simulink model "sampleModel106"  (R2022a)
settings: Solver=VariableStepAuto  StartTime=0.0  StopTime=10.0  RelTol=1e-3
undefined symbols (not defined in the file): DiscIntNeverNeededParam, magnitude, Newton, Raphson
libraries: simulink x379, slpidlib x89
(part 13 of 16)

== system sampleModel106/cfblk83/cfblk12/cfblk12/cfblk10 ==
  cfblk1 : Inport
  cfblk10 : Inport  Port=2
  cfblk11 : Inport  Port=3
  cfblk12 : Inport  Port=4
  cfblk13 : Inport  Port=5
  cfblk3 : DiscreteStateSpace
  cfblk4 : simulink/Discrete/Transfer Fcn Lead or Lag  PoleZ=0.95  ZeroZ=0.75  ICPrevOutput=0.0  ICPrevInput=0.0  DoSatur=off
      settings: SourceProductBaseCode=SL
  cfblk5 : ComplexToMagnitudeAngle
  cfblk6 : Reshape
  cfblk7 : PermuteDimensions
  cfblk8 : Signum
  cfblk9 : Constant  Value=[-735984474.100550]  SampleTime=1
  cfblk2 : Outport
  cfblk14 : Outport  Port=2
  cfblk15 : Outport  Port=3
  wires:
  cfblk6/1 -> cfblk8/1
  cfblk8/1 -> cfblk3/1
  cfblk5/1 -> cfblk15/1
  cfblk3/1 -> cfblk5/1
  cfblk10/1 -> cfblk7/1
  cfblk7/1 -> cfblk6/1
  cfblk13/1 -> cfblk4/1
  cfblk9/1 -> cfblk2/1
  cfblk12/1 -> cfblk14/1

== system sampleModel106/cfblk83/cfblk12/cfblk12/cfblk11 ==
  cfblk1 : Inport
  cfblk11 : Inport  Port=2
  cfblk12 : Inport  Port=3
  cfblk10 : Constant  Value=[-348173001.781500]  SampleTime=1
  cfblk3 : simulink/Discrete/Difference  ICPrevInput=0.0  OutMin=[]  OutMax=[]  OutDataTypeStr=Inherit: Inherit via back propagation  OutDataType=fixdt(1, 16)  OutScaling=2^-10  DoSatur=off
  cfblk4 : simulink/Discrete/Transfer Fcn First Order  PoleZ=0.95  ICPrevOutput=0.0  DoSatur=off
  cfblk5 : slpidlib/PID Controller  Controller=PID  Form=Parallel  TimeDomain=Discrete-time  UseExternalTs=off  SampleTime=1  IntegratorMethod=Forward Euler  FilterMethod=Forward Euler  ControllerParametersSource=internal  P=1  I=1  UseKiTs=off  D=0  N=100  UseFilter=on  TunerSelectOption=Transfer Function Based (PID Tuner App)  InitialConditionSource=internal  InitialConditionForIntegrator=0  InitialConditionForFilter=0  DifferentiatorICPrevScaledInput=0  ExternalReset=none  TrackingMode=off  Kt=1  LimitOutput=off  SatLimitsSource=internal  UpperSaturationLimit=inf  LowerSaturationLimit=-inf  LinearizeAsGain=off  AntiWindupMode=none  Kb=1  POutMin=[]  POutMax=[]  IOutMin=[]  IOutMax=[]  DOutMin=[]  DOutMax=[]  NOutMin=[]  NOutMax=[]  SumOutMin=[]  SumOutMax=[]  SaturationOutMin=[]  SaturationOutMax=[]  PParamMin=[]  PParamMax=[]  IParamMin=[]  IParamMax=[]  DParamMin=[]  DParamMax=[]  NParamMin=[]  NParamMax=[]  KbParamMin=[]  KbParamMax=[]  KtParamMin=[]  KtParamMax=[]  KbOutMin=[]  KbOutMax=[]  KtOutMin=[]  KtOutMax=[]  IntegratorOutMin=[]  IntegratorOutMax=[]  FilterOutMin=[]  FilterOutMax=[]  SumI1OutMin=[]  SumI1OutMax=[]  SumI2OutMin=[]  SumI2OutMax=[]  SumI3OutMin=[]  SumI3OutMax=[]  SumI4OutMin=[]  SumI4OutMax=[]  SumDOutMin=[]  SumDOutMax=[]  DifferentiatorOutMin=[]  DifferentiatorOutMax=[]  FilterDiffOutCoefMin=[]  FilterDiffOutCoefMax=[]  ReciprocalOutMin=[]  ReciprocalOutMax=[]  SumDenOutMin=[]  SumDenOutMax=[]  SumNumOutMin=[]  SumNumOutMax=[]  DivideOutMin=[]  DivideOutMax=[]  UdiffTsProdOutMin=[]  UdiffTsProdOutMax=[]  NTsProdOutMin=[]  NTsProdOutMax=[]  UintegralTsProdOutMin=[]  UintegralTsProdOutMax=[]  UngainTsProdOutMin=[]  UngainTsProdOutMax=[]  IntegratorContinuousStateAttributes=''  IntegratorStateMustResolveToSignalObject=off  IntegratorRTWStateStorageClass=Auto  FilterContinuousStateAttributes=''  FilterStateMustResolveToSignalObject=off  FilterRTWStateStorageClass=Auto  ParallelPVariant=InternalParameters  IdealPVariant=Disabled  IVariant=InternalParameters  DVariant=InternalParameters  IntegratorVariant=Discrete  SatVariant=Disabled  AWVariant=Passthrough  PCopyVariant=Disabled  TRVariant=Disabled  FdbkBlocksVariant=Forward  IdealPFdbkVariant=Disabled  SatFdbkVariant=Disabled  DerivativeFilterVariant=ForwardEulerFilter  NVariant=InternalParameters  NCopyVariant=Disabled  FilterICVariant=InternalICsFilter  IntegratorICVariant=InternalICs  ExternalResetVariant=Disabled  TRSumVariant=Passthrough  SumFdbkVariant=Disabled  SumVariant=Sum_PID  TsampFilterVariant=InternalTs  TsampNgainVariant=Passthrough  TsampIntegralVariant=Passthrough  ExternalSaturationOutDataTypeStr=Inherit: Same as second input  aMode=0
  cfblk6 : Rounding
  cfblk7 : Signum
  cfblk8 : Sqrt  Operator=rSqrt  AlgorithmType=Newton-Raphson
  cfblk9 : Constant  Value=[207257755.323865]  SampleTime=1
  cfblk2 : Outport
  wires:
  cfblk9/1 -> cfblk3/1
  cfblk7/1 -> cfblk2/1
  cfblk11/1 -> cfblk5/1
  cfblk10/1 -> cfblk7/1
  cfblk12/1 -> cfblk8/1
  cfblk6/1 -> cfblk4/1
  cfblk1/1 -> cfblk6/1

== system sampleModel106/cfblk83/cfblk12/cfblk13/cfblk10 ==
  cfblk1 : Inport
  cfblk10 : Sum  Inputs=--
  cfblk11 : Sin  TimeSource=Use external signal  SampleTime=0
  cfblk12 : Squeeze
  cfblk13 : Constant  Value=[-66310425.135306]  SampleTime=1
  cfblk14 : Constant  Value=[-311313699.679596]  SampleTime=1
  cfblk3 : DiscreteTransferFcn  SampleTime=1
  cfblk4 : slpidlib/PID Controller  Controller=PID  Form=Parallel  TimeDomain=Discrete-time  UseExternalTs=off  SampleTime=1  IntegratorMethod=Forward Euler  FilterMethod=Forward Euler  ControllerParametersSource=internal  P=1  I=1  UseKiTs=off  D=0  N=100  UseFilter=on  TunerSelectOption=Transfer Function Based (PID Tuner App)  InitialConditionSource=internal  InitialConditionForIntegrator=0  InitialConditionForFilter=0  DifferentiatorICPrevScaledInput=0  ExternalReset=none  TrackingMode=off  Kt=1  LimitOutput=off  SatLimitsSource=internal  UpperSaturationLimit=inf  LowerSaturationLimit=-inf  LinearizeAsGain=off  AntiWindupMode=none  Kb=1  POutMin=[]  POutMax=[]  IOutMin=[]  IOutMax=[]  DOutMin=[]  DOutMax=[]  NOutMin=[]  NOutMax=[]  SumOutMin=[]  SumOutMax=[]  SaturationOutMin=[]  SaturationOutMax=[]  PParamMin=[]  PParamMax=[]  IParamMin=[]  IParamMax=[]  DParamMin=[]  DParamMax=[]  NParamMin=[]  NParamMax=[]  KbParamMin=[]  KbParamMax=[]  KtParamMin=[]  KtParamMax=[]  KbOutMin=[]  KbOutMax=[]  KtOutMin=[]  KtOutMax=[]  IntegratorOutMin=[]  IntegratorOutMax=[]  FilterOutMin=[]  FilterOutMax=[]  SumI1OutMin=[]  SumI1OutMax=[]  SumI2OutMin=[]  SumI2OutMax=[]  SumI3OutMin=[]  SumI3OutMax=[]  SumI4OutMin=[]  SumI4OutMax=[]  SumDOutMin=[]  SumDOutMax=[]  DifferentiatorOutMin=[]  DifferentiatorOutMax=[]  FilterDiffOutCoefMin=[]  FilterDiffOutCoefMax=[]  ReciprocalOutMin=[]  ReciprocalOutMax=[]  SumDenOutMin=[]  SumDenOutMax=[]  SumNumOutMin=[]  SumNumOutMax=[]  DivideOutMin=[]  DivideOutMax=[]  UdiffTsProdOutMin=[]  UdiffTsProdOutMax=[]  NTsProdOutMin=[]  NTsProdOutMax=[]  UintegralTsProdOutMin=[]  UintegralTsProdOutMax=[]  UngainTsProdOutMin=[]  UngainTsProdOutMax=[]  IntegratorContinuousStateAttributes=''  IntegratorStateMustResolveToSignalObject=off  IntegratorRTWStateStorageClass=Auto  FilterContinuousStateAttributes=''  FilterStateMustResolveToSignalObject=off  FilterRTWStateStorageClass=Auto  ParallelPVariant=InternalParameters  IdealPVariant=Disabled  IVariant=InternalParameters  DVariant=InternalParameters  IntegratorVariant=Discrete  SatVariant=Disabled  AWVariant=Passthrough  PCopyVariant=Disabled  TRVariant=Disabled  FdbkBlocksVariant=Forward  IdealPFdbkVariant=Disabled  SatFdbkVariant=Disabled  DerivativeFilterVariant=ForwardEulerFilter  NVariant=InternalParameters  NCopyVariant=Disabled  FilterICVariant=InternalICsFilter  IntegratorICVariant=InternalICs  ExternalResetVariant=Disabled  TRSumVariant=Passthrough  SumFdbkVariant=Disabled  SumVariant=Sum_PID  TsampFilterVariant=InternalTs  TsampNgainVariant=Passthrough  TsampIntegralVariant=Passthrough  ExternalSaturationOutDataTypeStr=Inherit: Same as second input  aMode=0
  cfblk5 : simulink/Discrete/Transfer Fcn First Order  PoleZ=0.95  ICPrevOutput=0.0  DoSatur=off
  cfblk6 : Signum
  cfblk7 : Sum  Inputs=-+
  cfblk8 : UnaryMinus
  cfblk9 : Math  Operator=conj
  cfblk2 : Outport
  cfblk15 : Outport  Port=2
  cfblk16 : Outport  Port=3
  cfblk17 : Outport  Port=4
  wires:
  cfblk5/1 -> cfblk17/1
  cfblk7/1 -> cfblk15/1
  cfblk14/1 -> cfblk6/1
  cfblk13/1 -> cfblk4/1, cfblk11/1
  cfblk11/1 -> cfblk5/1, cfblk10/2
  cfblk1/1 -> cfblk10/1, cfblk9/1
  cfblk10/1 -> cfblk3/1
  cfblk9/1 -> cfblk7/1
  cfblk8/1 -> cfblk2/1
  cfblk6/1 -> cfblk7/2
  cfblk3/1 -> cfblk16/1
  cfblk4/1 -> cfblk12/1
  cfblk12/1 -> cfblk8/1

== system sampleModel106/cfblk83/cfblk12/cfblk13/cfblk8 ==
  cfblk1 : Inport
  cfblk13 : Inport  Port=2
  cfblk14 : Inport  Port=3
  cfblk10 : Constant  Value=[-221630629.444218]  SampleTime=1
  cfblk11 : Constant  Value=[651188913.954120]  SampleTime=1
  cfblk12 : Constant  Value=[-519214434.322099]  SampleTime=1
  cfblk3 : DiscreteTransferFcn  SampleTime=1
  cfblk4 : Delay  DelayLengthSource=Input port  SampleTime=1
      settings: InputPortMap=u0,p1
  cfblk5 : DiscreteFilter  SampleTime=1
  cfblk6 : slpidlib/PID Controller  Controller=PID  Form=Parallel  TimeDomain=Discrete-time  UseExternalTs=off  SampleTime=1  IntegratorMethod=Forward Euler  FilterMethod=Forward Euler  ControllerParametersSource=internal  P=1  I=1  UseKiTs=off  D=0  N=100  UseFilter=on  TunerSelectOption=Transfer Function Based (PID Tuner App)  InitialConditionSource=internal  InitialConditionForIntegrator=0  InitialConditionForFilter=0  DifferentiatorICPrevScaledInput=0  ExternalReset=none  TrackingMode=off  Kt=1  LimitOutput=off  SatLimitsSource=internal  UpperSaturationLimit=inf  LowerSaturationLimit=-inf  LinearizeAsGain=off  AntiWindupMode=none  Kb=1  POutMin=[]  POutMax=[]  IOutMin=[]  IOutMax=[]  DOutMin=[]  DOutMax=[]  NOutMin=[]  NOutMax=[]  SumOutMin=[]  SumOutMax=[]  SaturationOutMin=[]  SaturationOutMax=[]  PParamMin=[]  PParamMax=[]  IParamMin=[]  IParamMax=[]  DParamMin=[]  DParamMax=[]  NParamMin=[]  NParamMax=[]  KbParamMin=[]  KbParamMax=[]  KtParamMin=[]  KtParamMax=[]  KbOutMin=[]  KbOutMax=[]  KtOutMin=[]  KtOutMax=[]  IntegratorOutMin=[]  IntegratorOutMax=[]  FilterOutMin=[]  FilterOutMax=[]  SumI1OutMin=[]  SumI1OutMax=[]  SumI2OutMin=[]  SumI2OutMax=[]  SumI3OutMin=[]  SumI3OutMax=[]  SumI4OutMin=[]  SumI4OutMax=[]  SumDOutMin=[]  SumDOutMax=[]  DifferentiatorOutMin=[]  DifferentiatorOutMax=[]  FilterDiffOutCoefMin=[]  FilterDiffOutCoefMax=[]  ReciprocalOutMin=[]  ReciprocalOutMax=[]  SumDenOutMin=[]  SumDenOutMax=[]  SumNumOutMin=[]  SumNumOutMax=[]  DivideOutMin=[]  DivideOutMax=[]  UdiffTsProdOutMin=[]  UdiffTsProdOutMax=[]  NTsProdOutMin=[]  NTsProdOutMax=[]  UintegralTsProdOutMin=[]  UintegralTsProdOutMax=[]  UngainTsProdOutMin=[]  UngainTsProdOutMax=[]  IntegratorContinuousStateAttributes=''  IntegratorStateMustResolveToSignalObject=off  IntegratorRTWStateStorageClass=Auto  FilterContinuousStateAttributes=''  FilterStateMustResolveToSignalObject=off  FilterRTWStateStorageClass=Auto  ParallelPVariant=InternalParameters  IdealPVariant=Disabled  IVariant=InternalParameters  DVariant=InternalParameters  IntegratorVariant=Discrete  SatVariant=Disabled  AWVariant=Passthrough  PCopyVariant=Disabled  TRVariant=Disabled  FdbkBlocksVariant=Forward  IdealPFdbkVariant=Disabled  SatFdbkVariant=Disabled  DerivativeFilterVariant=ForwardEulerFilter  NVariant=InternalParameters  NCopyVariant=Disabled  FilterICVariant=InternalICsFilter  IntegratorICVariant=InternalICs  ExternalResetVariant=Disabled  TRSumVariant=Passthrough  SumFdbkVariant=Disabled  SumVariant=Sum_PID  TsampFilterVariant=InternalTs  TsampNgainVariant=Passthrough  TsampIntegralVariant=Passthrough  ExternalSaturationOutDataTypeStr=Inherit: Same as second input  aMode=0
  cfblk7 : Sum  Inputs=|++
  cfblk8 : DotProduct  OutDataTypeStr=Inherit: Inherit via internal rule
  cfblk9 : Constant  Value=[-97885654.836450]  SampleTime=1
  cfblk2 : Outport
  cfblk15 : Outport  Port=2
  cfblk16 : Outport  Port=3
  cfblk17 : Outport  Port=4
  wires:
  cfblk13/1 -> cfblk7/1
  cfblk9/1 -> cfblk5/1
  cfblk1/1 -> cfblk8/1
  cfblk11/1 -> cfblk7/2
  cfblk3/1 -> cfblk15/1
  cfblk7/1 -> cfblk8/2
  cfblk12/1 -> cfblk2/1
  cfblk14/1 -> cfblk16/1
  cfblk8/1 -> cfblk3/1
  cfblk4/1 -> cfblk17/1
  cfblk10/1 -> cfblk6/1
  cfblk6/1 -> cfblk4/1
  cfblk5/1 -> cfblk4/2

== system sampleModel106/cfblk83/cfblk12/cfblk13/cfblk9 ==
  cfblk1 : Inport
  cfblk13 : Inport  Port=2
  cfblk14 : Inport  Port=3
  cfblk15 : Inport  Port=4
  cfblk16 : Inport  Port=5
  cfblk10 : Product
  cfblk11 : Constant  Value=[-59332882.686168]  SampleTime=1
  cfblk12 : Constant  Value=[889332264.177902]  SampleTime=1
  cfblk3 : simulink/Discrete/Transfer Fcn Real Zero  ZeroZ=0.75  ICPrevInput=0.0  DoSatur=off
      settings: SourceProductBaseCode=SL
  cfblk4 : DiscreteStateSpace
  cfblk5 : Math  Operator=pow
  cfblk6 : Sum  Inputs=+
  cfblk7 : Squeeze
  cfblk8 : Sum  Inputs=+-
  cfblk9 : Reshape
  cfblk2 : Outport
  cfblk17 : Outport  Port=2
  wires:
  cfblk13/1 -> cfblk4/1
  cfblk8/1 -> cfblk6/1
  cfblk9/1 -> cfblk17/1
  cfblk4/1 -> cfblk8/1
  cfblk7/1 -> cfblk3/1
  cfblk11/1 -> cfblk9/1
  cfblk16/1 -> cfblk5/1
  cfblk1/1 -> cfblk5/2
  cfblk12/1 -> cfblk2/1
  cfblk15/1 -> cfblk7/1
  cfblk5/1 -> cfblk8/2
  cfblk14/1 -> cfblk10/1
  cfblk6/1 -> cfblk10/2

== system sampleModel106/cfblk83/cfblk13/cfblk11/cfblk9 ==
  cfblk1 : Inport
  cfblk12 : Inport  Port=2
  cfblk10 : Constant  Value=[979832863.962545]  SampleTime=1
  cfblk11 : Constant  Value=[551392504.886462]  SampleTime=1
  cfblk14 : Delay  SampleTime=1
  cfblk3 : Sum  Inputs=+
  cfblk4 : Assignment  DiagnosticForDimensions=Warning  IndexOptions=Index vector (dialog)  Indices=1  OutputSizes=1
  cfblk5 : Sqrt
  cfblk6 : Sqrt  Operator=rSqrt  AlgorithmType=Newton-Raphson
  cfblk7 : Squeeze
  cfblk8 : Constant  Value=[798337658.700192]  SampleTime=1
  cfblk9 : Constant  Value=[-485920315.300231]  SampleTime=1
  cfblk2 : Outport
  cfblk13 : Outport  Port=2
  wires:
  cfblk11/1 -> cfblk7/1
  cfblk7/1 -> cfblk13/1
  cfblk9/1 -> cfblk5/1
  cfblk10/1 -> cfblk6/1
  cfblk1/1 -> cfblk2/1
  cfblk8/1 -> cfblk4/1
  cfblk3/1 -> cfblk4/2
  cfblk4/1 -> cfblk14/1
  cfblk14/1 -> cfblk3/1

== system sampleModel106/cfblk83/cfblk13/cfblk12/cfblk5 ==
  cfblk1 : Inport
  cfblk11 : Inport  Port=2
  cfblk12 : Inport  Port=3
  cfblk13 : Inport  Port=4
  cfblk14 : Inport  Port=5
  cfblk15 : Inport  Port=6
  cfblk16 : Inport  Port=7
  cfblk10 : Constant  Value=[611025124.323310]  SampleTime=1
  cfblk18 : Delay  SampleTime=1
  cfblk3 : Delay  ShowEnablePort=on  SampleTime=1
      settings: InputPortMap=u0,e6
  cfblk4 : Sum  Inputs=-+
  cfblk5 : Signum
  cfblk6 : Product
  cfblk7 : ComplexToMagnitudeAngle
  cfblk8 : DotProduct  OutDataTypeStr=Inherit: Inherit via internal rule
  cfblk9 : Assignment  DiagnosticForDimensions=Warning  IndexOptions=Index vector (dialog)  Indices=1  OutputSizes=1
  cfblk2 : Outport
  cfblk17 : Outport  Port=2
  wires:
  cfblk15/1 -> cfblk3/1
  cfblk5/1 -> cfblk7/1
  cfblk6/1 -> cfblk4/1
  cfblk1/1 -> cfblk3/2
  cfblk8/1 -> cfblk2/1
  cfblk12/1 -> cfblk8/1
  cfblk13/1 -> cfblk17/1
  cfblk16/1 -> cfblk5/1
  cfblk10/1 -> cfblk4/2
  cfblk11/1 -> cfblk9/1
  cfblk3/1 -> cfblk6/2
  cfblk7/1 -> cfblk8/2
  cfblk4/1 -> cfblk9/2
  cfblk9/1 -> cfblk18/1
  cfblk18/1 -> cfblk6/1

== system sampleModel106/cfblk83/cfblk13/cfblk12/cfblk6 ==
  cfblk1 : Inport
  cfblk10 : Gain  Gain=[293098853.914123]
  cfblk11 : Gain  Gain=[-612575929.200624]
  cfblk12 : Gain  Gain=[945578202.855884]
  cfblk13 : Constant  Value=[-519498832.994828]  SampleTime=1
  cfblk16 : Delay  SampleTime=1
  cfblk3 : Delay  DelayLengthSource=Input port  SampleTime=1
      settings: InputPortMap=u0,p1
  cfblk4 : simulink/Discrete/Difference  ICPrevInput=0.0  OutMin=[]  OutMax=[]  OutDataTypeStr=Inherit: Inherit via back propagation  OutDataType=fixdt(1, 16)  OutScaling=2^-10  DoSatur=off
  cfblk5 : Delay  ShowEnablePort=on  SampleTime=1
      settings: InputPortMap=u0,e6
  cfblk6 : UnitDelay  HasFrameUpgradeWarning=on
  cfblk7 : Rounding
  cfblk8 : MinMax  Function=max
  cfblk9 : Polyval  Coefs=[ +2.081618890e-019, -1.441693666e-014, +4.719686976e-010, -8.536869453e-006, +1.621573104e-001, -8.087801117e+001 ]
  cfblk2 : Outport
  cfblk14 : Outport  Port=2
  cfblk15 : Outport  Port=3
  wires:
  cfblk6/1 -> cfblk9/1
  cfblk12/1 -> cfblk14/1
  cfblk1/1 -> cfblk3/1
  cfblk9/1 -> cfblk15/1, cfblk5/2
  cfblk7/1 -> cfblk6/1
  cfblk3/1 -> cfblk8/1
  cfblk10/1 -> cfblk7/1
  cfblk4/1 -> cfblk5/1
  cfblk8/1 -> cfblk11/1, cfblk12/1
  cfblk13/1 -> cfblk2/1, cfblk10/1
  cfblk11/1 -> cfblk4/1
  cfblk5/1 -> cfblk16/1
  cfblk16/1 -> cfblk3/2

== system sampleModel106/cfblk83/cfblk13/cfblk12/cfblk7 ==
  cfblk1 : Inport
  cfblk12 : Inport  Port=2
  cfblk13 : Inport  Port=3
  cfblk14 : Inport  Port=4
  cfblk15 : Inport  Port=5
  cfblk10 : Constant  Value=[931392199.249037]  SampleTime=1
  cfblk11 : Constant  Value=[718235558.917173]  SampleTime=1
  cfblk3 : Delay  SampleTime=1
  cfblk4 : DiscreteFilter  SampleTime=1
  cfblk5 : Rounding
  cfblk6 : DotProduct  OutDataTypeStr=Inherit: Inherit via internal rule
  cfblk7 : UnaryMinus
  cfblk8 : Trigonometry
  cfblk9 : Squeeze
  cfblk2 : Outport
  cfblk16 : Outport  Port=2
  wires:
  cfblk11/1 -> cfblk6/1
  cfblk5/1 -> cfblk4/1
  cfblk6/1 -> cfblk7/1
  cfblk14/1 -> cfblk5/1
  cfblk12/1 -> cfblk6/2
  cfblk13/1 -> cfblk9/1
  cfblk9/1 -> cfblk2/1
  cfblk15/1 -> cfblk3/1
  cfblk7/1 -> cfblk16/1
  cfblk3/1 -> cfblk8/1

== system sampleModel106/cfblk83/cfblk13/cfblk12/cfblk8 ==
  cfblk1 : Inport
  cfblk7 : Inport  Port=2
  cfblk8 : Inport  Port=3
  cfblk3 : Abs  SaturateOnIntegerOverflow=off
  cfblk4 : ComplexToMagnitudeAngle
  cfblk5 : Sum  Inputs=|++
  cfblk6 : Squeeze
  cfblk2 : Outport
  wires:
  cfblk5/1 -> cfblk2/1
  cfblk4/1 -> cfblk6/1
  cfblk1/1 -> cfblk5/1
  cfblk8/1 -> cfblk3/1
  cfblk6/1 -> cfblk5/2
  cfblk7/1 -> cfblk4/1

== system sampleModel106/cfblk83/cfblk13/cfblk13/cfblk8 ==
  cfblk1 : Inport
  cfblk10 : Inport  Port=2
  cfblk11 : Inport  Port=3
  cfblk3 : Trigonometry
  cfblk4 : Trigonometry
  cfblk5 : Trigonometry
  cfblk6 : Sin  TimeSource=Use external signal  SampleTime=0
  cfblk7 : Squeeze
  cfblk8 : Sum  Inputs=|++
  cfblk9 : Constant  Value=[938603763.562760]  SampleTime=1
  cfblk2 : Outport
  cfblk12 : Outport  Port=2
  wires:
  cfblk4/1 -> cfblk8/1
  cfblk3/1 -> cfblk6/1
  cfblk9/1 -> cfblk4/1
  cfblk6/1 -> cfblk12/1
  cfblk1/1 -> cfblk8/2
  cfblk11/1 -> cfblk5/1
  cfblk5/1 -> cfblk3/1
  cfblk10/1 -> cfblk7/1
  cfblk8/1 -> cfblk2/1

== system sampleModel106/cfblk83/cfblk13/cfblk13/cfblk9 ==
  cfblk1 : Inport
  cfblk11 : Inport  Port=2
  cfblk10 : Constant  Value=[825217161.468918]  SampleTime=1
  cfblk13 : Delay  SampleTime=1
  cfblk3 : UnitDelay  HasFrameUpgradeWarning=on
  cfblk4 : UnitDelay  HasFrameUpgradeWarning=on
  cfblk5 : DiscreteFir  SampleTime=1
  cfblk6 : simulink/Discrete/Transfer Fcn First Order  PoleZ=0.95  ICPrevOutput=0.0  DoSatur=off
  cfblk7 : ComplexToMagnitudeAngle
  cfblk8 : Sum  Inputs=+
  cfblk9 : Constant  Value=[262988150.516446]  SampleTime=1
  cfblk2 : Outport
  cfblk12 : Outport  Port=2
  wires:
  cfblk8/1 -> cfblk6/1
  cfblk10/1 -> cfblk8/1
  cfblk1/1 -> cfblk2/1
  cfblk9/1 -> cfblk12/1
  cfblk3/1 -> cfblk7/1
  cfblk7/1 -> cfblk4/1
  cfblk7/2 -> cfblk5/1
  cfblk4/1 -> cfblk13/1
  cfblk13/1 -> cfblk3/1

== system sampleModel106/cfblk84/cfblk10/cfblk10/cfblk10 ==
  cfblk1 : Inport
  cfblk6 : Inport  Port=2
  cfblk3 : UnitDelay  SampleTime=-1  HasFrameUpgradeWarning=on
  cfblk4 : Product  Inputs=*
  cfblk5 : DotProduct  OutDataTypeStr=Inherit: Inherit via internal rule
  cfblk2 : Outport
  cfblk7 : Outport  Port=2
  wires:
  cfblk4/1 -> cfblk2/1
  cfblk3/1 -> cfblk4/1, cfblk5/2
  cfblk6/1 -> cfblk3/1
  cfblk5/1 -> cfblk7/1
  cfblk1/1 -> cfblk5/1

== system sampleModel106/cfblk84/cfblk10/cfblk10/cfblk11 ==
  cfblk1 : Inport
  cfblk7 : Inport  Port=2
  cfblk3 : DiscreteFilter
  cfblk4 : Sum  Inputs=|++
  cfblk5 : Product  Inputs=*
  cfblk6 : Sqrt  Operator=rSqrt  AlgorithmType=Newton-Raphson
  cfblk2 : Outport
  cfblk8 : Outport  Port=2
  wires:
  cfblk7/1 -> cfblk3/1
  cfblk6/1 -> cfblk4/1
  cfblk3/1 -> cfblk8/1
  cfblk5/1 -> cfblk2/1
  cfblk1/1 -> cfblk4/2, cfblk6/1
  cfblk4/1 -> cfblk5/1

== system sampleModel106/cfblk84/cfblk10/cfblk8/cfblk8 ==
  cfblk1 : Inport
  cfblk11 : Delay
  cfblk12 : Delay
  cfblk3 : DiscreteFilter
  cfblk4 : simulink/Discrete/Difference  ICPrevInput=0.0  OutMin=[]  OutMax=[]  OutDataTypeStr=Inherit: Inherit via back propagation  OutDataType=fixdt(1, 16)  OutScaling=2^-10  DoSatur=off
  cfblk5 : DotProduct  OutDataTypeStr=Inherit: Inherit via internal rule
  cfblk6 : UnaryMinus
  cfblk7 : Squeeze
  cfblk2 : Outport
  cfblk8 : Outport  Port=2
  cfblk9 : Outport  Port=3
  cfblk10 : Outport  Port=4
  wires:
  cfblk1/1 -> cfblk9/1, cfblk7/1
  cfblk7/1 -> cfblk10/1
  cfblk5/1 -> cfblk6/1, cfblk3/1, cfblk8/1
  cfblk4/1 -> cfblk2/1
  cfblk6/1 -> cfblk11/1, cfblk12/1
  cfblk3/1 -> cfblk4/1
  cfblk11/1 -> cfblk5/1
  cfblk12/1 -> cfblk5/2

== system sampleModel106/cfblk84/cfblk10/cfblk9/cfblk5 ==
  cfblk1 : Inport
  cfblk6 : Inport  Port=2
  cfblk7 : Inport  Port=3
  cfblk3 : Sum  Inputs=+-
  cfblk4 : Polyval  Coefs=[ +2.081618890e-019, -1.441693666e-014, +4.719686976e-010, -8.536869453e-006, +1.621573104e-001, -8.087801117e+001 ]
  cfblk5 : Constant  Value=[-658032411.007219]  SampleTime=1
  cfblk2 : Outport
  wires:
  cfblk5/1 -> cfblk4/1
  cfblk3/1 -> cfblk2/1
  cfblk7/1 -> cfblk3/1
  cfblk4/1 -> cfblk3/2

== system sampleModel106/cfblk84/cfblk10/cfblk9/cfblk6 ==
  cfblk1 : Inport
  cfblk9 : Inport  Port=2
  cfblk10 : Inport  Port=3
  cfblk11 : Inport  Port=4
  cfblk12 : Inport  Port=5
  cfblk3 : slpidlib/PID Controller (2DOF)  Controller=PID  Form=Parallel  TimeDomain=Discrete-time  UseExternalTs=off  SampleTime=-1  IntegratorMethod=Forward Euler  FilterMethod=Forward Euler  ControllerParametersSource=internal  P=1  I=1  UseKiTs=off  D=0  N=100  UseFilter=on  b=1  c=1  TunerSelectOption=Transfer Function Based (PID Tuner App)  InitialConditionSource=internal  InitialConditionForIntegrator=0  InitialConditionForFilter=0  DifferentiatorICPrevScaledInput=0  ExternalReset=none  TrackingMode=off  Kt=1  LimitOutput=off  SatLimitsSource=internal  UpperSaturationLimit=inf  LowerSaturationLimit=-inf  LinearizeAsGain=off  AntiWindupMode=none  Kb=1  POutMin=[]  POutMax=[]  IOutMin=[]  IOutMax=[]  DOutMin=[]  DOutMax=[]  NOutMin=[]  NOutMax=[]  bOutMin=[]  bOutMax=[]  cOutMin=[]  cOutMax=[]  SumOutMin=[]  SumOutMax=[]  SaturationOutMin=[]  SaturationOutMax=[]  PParamMin=[]  PParamMax=[]  IParamMin=[]  IParamMax=[]  DParamMin=[]  DParamMax=[]  NParamMin=[]  NParamMax=[]  bParamMin=[]  bParamMax=[]  cParamMin=[]  cParamMax=[]  KbParamMin=[]  KbParamMax=[]  KtParamMin=[]  KtParamMax=[]  KbOutMin=[]  KbOutMax=[]  KtOutMin=[]  KtOutMax=[]  IntegratorOutMin=[]  IntegratorOutMax=[]  FilterOutMin=[]  FilterOutMax=[]  SumI1OutMin=[]  SumI1OutMax=[]  SumI2OutMin=[]  SumI2OutMax=[]  SumI3OutMin=[]  SumI3OutMax=[]  SumI4OutMin=[]  SumI4OutMax=[]  SumDOutMin=[]  SumDOutMax=[]  Sum1OutMin=[]  Sum1OutMax=[]  Sum2OutMin=[]  Sum2OutMax=[]  Sum3OutMin=[]  Sum3OutMax=[]  DifferentiatorOutMin=[]  DifferentiatorOutMax=[]  FilterDiffOutCoefMin=[]  FilterDiffOutCoefMax=[]  ReciprocalOutMin=[]  ReciprocalOutMax=[]  SumDenOutMin=[]  SumDenOutMax=[]  SumNumOutMin=[]  SumNumOutMax=[]  DivideOutMin=[]  DivideOutMax=[]  UdiffTsProdOutMin=[]  UdiffTsProdOutMax=[]  NTsProdOutMin=[]  NTsProdOutMax=[]  UintegralTsProdOutMin=[]  UintegralTsProdOutMax=[]  UngainTsProdOutMin=[]  UngainTsProdOutMax=[]  IntegratorContinuousStateAttributes=''  IntegratorStateMustResolveToSignalObject=off  IntegratorRTWStateStorageClass=Auto  FilterContinuousStateAttributes=''  FilterStateMustResolveToSignalObject=off  FilterRTWStateStorageClass=Auto  ParallelPVariant=InternalParameters  IdealPVariant=Disabled  IVariant=InternalParameters  DVariant=InternalParameters  bVariant=InternalParameters  cVariant=InternalParameters  IntegratorVariant=Discrete  SatVariant=Disabled  AWVariant=Passthrough  PCopyVariant=Disabled  TRVariant=Disabled  FdbkBlocksVariant=Forward  IdealPFdbkVariant=Disabled  SatFdbkVariant=Disabled  DerivativeFilterVariant=ForwardEulerFilter  NVariant=InternalParameters  NCopyVariant=Disabled  FilterICVariant=InternalICsFilter  IntegratorICVariant=InternalICs  ExternalResetVariant=Disabled  TRSumVariant=Passthrough  SumFdbkVariant=Disabled  SumVariant=Sum_PID  TsampFilterVariant=InternalTs  TsampNgainVariant=Passthrough  TsampIntegralVariant=Passthrough  ExternalSaturationOutDataTypeStr=Inherit: Same as second input
      settings: SourceProductBaseCode=SL
  cfblk4 : Product  Inputs=**
  cfblk5 : Abs  SaturateOnIntegerOverflow=off
  cfblk6 : Math  Operator=log
  cfblk7 : Constant  Value=[896531267.897951]  SampleTime=1
  cfblk8 : Constant  Value=[637844265.256375]  SampleTime=1
  cfblk2 : Outport
  wires:
  cfblk3/1 -> cfblk5/1
  cfblk12/1 -> cfblk6/1
  cfblk1/1 -> cfblk4/1
  cfblk9/1 -> cfblk4/2
  cfblk7/1 -> cfblk2/1
  cfblk11/1 -> cfblk3/1
  cfblk8/1 -> cfblk3/2

== system sampleModel106/cfblk84/cfblk5/cfblk13/cfblk10 ==
  cfblk1 : Inport
  cfblk10 : Constant  Value=[-863173645.416676]  SampleTime=1
  cfblk11 : Constant  Value=[-99275692.541480]  SampleTime=1
  cfblk14 : Delay  SampleTime=1
  cfblk3 : simulink/Discrete/Tapped Delay  vinit=0.0  samptime=-1  NumDelays=1  DelayOrder=Oldest  includeCurrent=off
  cfblk4 : simulink/Discrete/Difference  ICPrevInput=0.0  OutMin=[]  OutMax=[]  OutDataTypeStr=Inherit: Inherit via back propagation  OutDataType=fixdt(1, 16)  OutScaling=2^-10  DoSatur=off
  cfblk5 : Delay  SampleTime=1
  cfblk6 : DotProduct  OutDataTypeStr=Inherit: Inherit via internal rule
  cfblk7 : Sqrt  Operator=rSqrt  AlgorithmType=Newton-Raphson
  cfblk8 : Sum  Inputs=+
  cfblk9 : Constant  Value=[477108463.607855]  SampleTime=1
  cfblk2 : Outport
  cfblk12 : Outport  Port=2
  cfblk13 : Outport  Port=3
  wires:
  cfblk4/1 -> cfblk5/1
  cfblk10/1 -> cfblk7/1
  cfblk6/1 -> cfblk4/1
  cfblk7/1 -> cfblk6/1
  cfblk3/1 -> cfblk6/2
  cfblk11/1 -> cfblk12/1
  cfblk1/1 -> cfblk8/1
  cfblk8/1 -> cfblk13/1
  cfblk9/1 -> cfblk2/1
  cfblk5/1 -> cfblk14/1
  cfblk14/1 -> cfblk3/1

== system sampleModel106/cfblk84/cfblk5/cfblk13/cfblk11 ==
  cfblk1 : Inport
  cfblk7 : Inport  Port=2
  cfblk8 : Inport  Port=3
  cfblk3 : simulink/Discrete/Transfer Fcn Real Zero  ZeroZ=0.75  ICPrevInput=0.0  DoSatur=off
      settings: SourceProductBaseCode=SL
  cfblk4 : Math  Operator=hypot
  cfblk5 : Constant  Value=[465220833.112546]  SampleTime=1
  cfblk6 : Constant  Value=[440580258.733231]  SampleTime=1
  cfblk2 : Outport
  cfblk9 : Outport  Port=2
  cfblk10 : Outport  Port=3
  cfblk11 : Outport  Port=4
  wires:
  cfblk4/1 -> cfblk9/1
  cfblk7/1 -> cfblk3/1
  cfblk6/1 -> cfblk2/1
  cfblk8/1 -> cfblk10/1
  cfblk3/1 -> cfblk11/1
  cfblk5/1 -> cfblk4/1
  cfblk1/1 -> cfblk4/2

== system sampleModel106/cfblk84/cfblk5/cfblk13/cfblk12 ==
  cfblk1 : Inport
  cfblk11 : Inport  Port=2
  cfblk12 : Inport  Port=3
  cfblk13 : Inport  Port=4
  cfblk14 : Inport  Port=5
  cfblk10 : Constant  Value=[536671838.031221]  SampleTime=1
  cfblk3 : simulink/Discrete/Transfer Fcn Real Zero  ZeroZ=0.75  ICPrevInput=0.0  DoSatur=off
      settings: SourceProductBaseCode=SL
  cfblk4 : PermuteDimensions
  cfblk5 : Sum  Inputs=+
  cfblk6 : Sqrt  Operator=rSqrt  AlgorithmType=Newton-Raphson
  cfblk7 : Squeeze
  cfblk8 : Constant  Value=[-734815010.273038]  SampleTime=1
  cfblk9 : Constant  Value=[-658292336.627287]  SampleTime=1
  cfblk2 : Outport
  wires:
  cfblk6/1 -> cfblk5/1
  cfblk7/1 -> cfblk3/1
  cfblk13/1 -> cfblk4/1
  cfblk11/1 -> cfblk6/1
  cfblk4/1 -> cfblk2/1
  cfblk1/1 -> cfblk7/1

== system sampleModel106/cfblk84/cfblk5/cfblk13/cfblk13 ==
  cfblk1 : Inport
  cfblk9 : Inport  Port=2
  cfblk3 : simulink/Discrete/Tapped Delay  vinit=0.0  samptime=-1  NumDelays=1  DelayOrder=Oldest  includeCurrent=off
  cfblk4 : UnaryMinus
  cfblk5 : MinMax  Function=max  Inputs=2
  cfblk6 : Squeeze
  cfblk7 : Constant  Value=[-716204746.836995]  SampleTime=1
  cfblk8 : Constant  Value=[824785440.207083]  SampleTime=1
  cfblk2 : Outport
  cfblk10 : Outport  Port=2
  wires:
  cfblk8/1 -> cfblk3/1
  cfblk6/1 -> cfblk2/1
  cfblk9/1 -> cfblk4/1
  cfblk4/1 -> cfblk10/1
  cfblk7/1 -> cfblk5/1
  cfblk1/1 -> cfblk6/1
  cfblk3/1 -> cfblk5/2

== system sampleModel106/cfblk84/cfblk5/cfblk13/cfblk18 ==
  cfblk1 : Inport
  cfblk14 : Inport  Port=2
  cfblk15 : Inport  Port=3
  cfblk16 : Inport  Port=4
  Action Port : ActionPort  ActionPortLabel=if(u1 >= 0)
  cfblk10 : Rounding
  cfblk11 : Constant  Value=[-558026556.463259]  SampleTime=1
  cfblk12 : Constant  Value=[225158940.621101]  SampleTime=1
  cfblk13 : Constant  Value=[599969272.968236]  SampleTime=1
  cfblk3 : DiscreteFilter
  cfblk4 : DiscreteStateSpace  SampleTime=-1
  cfblk5 : simulink/Discrete/Transfer Fcn Lead or Lag  PoleZ=0.95  ZeroZ=0.75  ICPrevOutput=0.0  ICPrevInput=0.0  DoSatur=off
      settings: SourceProductBaseCode=SL
  cfblk6 : slpidlib/PID Controller (2DOF)  Controller=PID  Form=Parallel  TimeDomain=Discrete-time  UseExternalTs=off  SampleTime=-1  IntegratorMethod=Forward Euler  FilterMethod=Forward Euler  ControllerParametersSource=internal  P=1  I=1  UseKiTs=off  D=0  N=100  UseFilter=on  b=1  c=1  TunerSelectOption=Transfer Function Based (PID Tuner App)  InitialConditionSource=internal  InitialConditionForIntegrator=0  InitialConditionForFilter=0  DifferentiatorICPrevScaledInput=0  ExternalReset=none  TrackingMode=off  Kt=1  LimitOutput=off  SatLimitsSource=internal  UpperSaturationLimit=inf  LowerSaturationLimit=-inf  LinearizeAsGain=off  AntiWindupMode=none  Kb=1  POutMin=[]  POutMax=[]  IOutMin=[]  IOutMax=[]  DOutMin=[]  DOutMax=[]  NOutMin=[]  NOutMax=[]  bOutMin=[]  bOutMax=[]  cOutMin=[]  cOutMax=[]  SumOutMin=[]  SumOutMax=[]  SaturationOutMin=[]  SaturationOutMax=[]  PParamMin=[]  PParamMax=[]  IParamMin=[]  IParamMax=[]  DParamMin=[]  DParamMax=[]  NParamMin=[]  NParamMax=[]  bParamMin=[]  bParamMax=[]  cParamMin=[]  cParamMax=[]  KbParamMin=[]  KbParamMax=[]  KtParamMin=[]  KtParamMax=[]  KbOutMin=[]  KbOutMax=[]  KtOutMin=[]  KtOutMax=[]  IntegratorOutMin=[]  IntegratorOutMax=[]  FilterOutMin=[]  FilterOutMax=[]  SumI1OutMin=[]  SumI1OutMax=[]  SumI2OutMin=[]  SumI2OutMax=[]  SumI3OutMin=[]  SumI3OutMax=[]  SumI4OutMin=[]  SumI4OutMax=[]  SumDOutMin=[]  SumDOutMax=[]  Sum1OutMin=[]  Sum1OutMax=[]  Sum2OutMin=[]  Sum2OutMax=[]  Sum3OutMin=[]  Sum3OutMax=[]  DifferentiatorOutMin=[]  DifferentiatorOutMax=[]  FilterDiffOutCoefMin=[]  FilterDiffOutCoefMax=[]  ReciprocalOutMin=[]  ReciprocalOutMax=[]  SumDenOutMin=[]  SumDenOutMax=[]  SumNumOutMin=[]  SumNumOutMax=[]  DivideOutMin=[]  DivideOutMax=[]  UdiffTsProdOutMin=[]  UdiffTsProdOutMax=[]  NTsProdOutMin=[]  NTsProdOutMax=[]  UintegralTsProdOutMin=[]  UintegralTsProdOutMax=[]  UngainTsProdOutMin=[]  UngainTsProdOutMax=[]  IntegratorContinuousStateAttributes=''  IntegratorStateMustResolveToSignalObject=off  IntegratorRTWStateStorageClass=Auto  FilterContinuousStateAttributes=''  FilterStateMustResolveToSignalObject=off  FilterRTWStateStorageClass=Auto  ParallelPVariant=InternalParameters  IdealPVariant=Disabled  IVariant=InternalParameters  DVariant=InternalParameters  bVariant=InternalParameters  cVariant=InternalParameters  IntegratorVariant=Discrete  SatVariant=Disabled  AWVariant=Passthrough  PCopyVariant=Disabled  TRVariant=Disabled  FdbkBlocksVariant=Forward  IdealPFdbkVariant=Disabled  SatFdbkVariant=Disabled  DerivativeFilterVariant=ForwardEulerFilter  NVariant=InternalParameters  NCopyVariant=Disabled  FilterICVariant=InternalICsFilter  IntegratorICVariant=InternalICs  ExternalResetVariant=Disabled  TRSumVariant=Passthrough  SumFdbkVariant=Disabled  SumVariant=Sum_PID  TsampFilterVariant=InternalTs  TsampNgainVariant=Passthrough  TsampIntegralVariant=Passthrough  ExternalSaturationOutDataTypeStr=Inherit: Same as second input
      settings: SourceProductBaseCode=SL
  cfblk7 : DiscreteIntegrator  SampleTime=-1  ICPrevOutput=DiscIntNeverNeededParam  ICPrevScaledInput=DiscIntNeverNeededParam
  cfblk8 : Sum  Inputs=+-
  cfblk9 : Product
  cfblk2 : Outport
  cfblk17 : Outport  Port=2
  wires:
  cfblk7/1 -> cfblk3/1
  cfblk6/1 -> cfblk4/1
  cfblk5/1 -> cfblk2/1
  cfblk8/1 -> cfblk7/1
  cfblk9/1 -> cfblk8/1
  cfblk10/1 -> cfblk8/2
  cfblk4/1 -> cfblk9/1
  cfblk13/1 -> cfblk9/2
  cfblk15/1 -> cfblk17/1
  cfblk11/1 -> cfblk10/1
  cfblk14/1 -> cfblk5/1
  cfblk1/1 -> cfblk6/1
  cfblk16/1 -> cfblk6/2

== system sampleModel106/cfblk84/cfblk5/cfblk13/cfblk19 ==
  cfblk1 : Inport
  cfblk11 : Inport  Port=2
  cfblk12 : Inport  Port=3
  cfblk13 : Inport  Port=4
  Action Port : ActionPort  ActionPortLabel=else
  cfblk10 : Constant  Value=[-821131582.178781]  SampleTime=1
  cfblk14 : Delay
  cfblk3 : Delay  ShowEnablePort=on
      settings: InputPortMap=u0,e6
  cfblk4 : Product  Inputs=**
  cfblk5 : Product  Inputs=**
  cfblk6 : Sin  TimeSource=Use external signal  SampleTime=0
  cfblk7 : Trigonometry
  cfblk8 : Assignment  DiagnosticForDimensions=Warning  IndexOptions=Index vector (dialog)  Indices=1  OutputSizes=1
  cfblk9 : Constant  Value=[-695021795.884194]  SampleTime=1
  cfblk2 : Outport
  wires:
  cfblk12/1 -> cfblk2/1
  cfblk10/1 -> cfblk6/1
  cfblk9/1 -> cfblk3/1
  cfblk1/1 -> cfblk3/2
  cfblk3/1 -> cfblk8/1
  cfblk13/1 -> cfblk8/2
  cfblk11/1 -> cfblk4/1
  cfblk6/1 -> cfblk7/1
  cfblk8/1 -> cfblk5/1
  cfblk5/1 -> cfblk4/2
  cfblk4/1 -> cfblk14/1
  cfblk14/1 -> cfblk5/2

== system sampleModel106/cfblk84/cfblk5/cfblk13/cfblk8 ==
  cfblk1 : Inport
  cfblk16 : Inport  Port=2
  cfblk17 : Inport  Port=3
  cfblk10 : Sum  Inputs=|++
  cfblk11 : Assignment  DiagnosticForDimensions=Warning  IndexOptions=Index vector (dialog)  Indices=1  OutputSizes=1
  cfblk12 : PermuteDimensions
  cfblk13 : Constant  Value=[942830516.653013]  SampleTime=1
  cfblk14 : Constant  Value=[603073261.025064]  SampleTime=1
  cfblk15 : Constant  Value=[-748654700.957018]  SampleTime=1
  cfblk3 : DiscreteTransferFcn  SampleTime=1
  cfblk4 : slpidlib/PID Controller  Controller=PID  Form=Parallel  TimeDomain=Discrete-time  UseExternalTs=off  SampleTime=1  IntegratorMethod=Forward Euler  FilterMethod=Forward Euler  ControllerParametersSource=internal  P=1  I=1  UseKiTs=off  D=0  N=100  UseFilter=on  TunerSelectOption=Transfer Function Based (PID Tuner App)  InitialConditionSource=internal  InitialConditionForIntegrator=0  InitialConditionForFilter=0  DifferentiatorICPrevScaledInput=0  ExternalReset=none  TrackingMode=off  Kt=1  LimitOutput=off  SatLimitsSource=internal  UpperSaturationLimit=inf  LowerSaturationLimit=-inf  LinearizeAsGain=off  AntiWindupMode=none  Kb=1  POutMin=[]  POutMax=[]  IOutMin=[]  IOutMax=[]  DOutMin=[]  DOutMax=[]  NOutMin=[]  NOutMax=[]  SumOutMin=[]  SumOutMax=[]  SaturationOutMin=[]  SaturationOutMax=[]  PParamMin=[]  PParamMax=[]  IParamMin=[]  IParamMax=[]  DParamMin=[]  DParamMax=[]  NParamMin=[]  NParamMax=[]  KbParamMin=[]  KbParamMax=[]  KtParamMin=[]  KtParamMax=[]  KbOutMin=[]  KbOutMax=[]  KtOutMin=[]  KtOutMax=[]  IntegratorOutMin=[]  IntegratorOutMax=[]  FilterOutMin=[]  FilterOutMax=[]  SumI1OutMin=[]  SumI1OutMax=[]  SumI2OutMin=[]  SumI2OutMax=[]  SumI3OutMin=[]  SumI3OutMax=[]  SumI4OutMin=[]  SumI4OutMax=[]  SumDOutMin=[]  SumDOutMax=[]  DifferentiatorOutMin=[]  DifferentiatorOutMax=[]  FilterDiffOutCoefMin=[]  FilterDiffOutCoefMax=[]  ReciprocalOutMin=[]  ReciprocalOutMax=[]  SumDenOutMin=[]  SumDenOutMax=[]  SumNumOutMin=[]  SumNumOutMax=[]  DivideOutMin=[]  DivideOutMax=[]  UdiffTsProdOutMin=[]  UdiffTsProdOutMax=[]  NTsProdOutMin=[]  NTsProdOutMax=[]  UintegralTsProdOutMin=[]  UintegralTsProdOutMax=[]  UngainTsProdOutMin=[]  UngainTsProdOutMax=[]  IntegratorContinuousStateAttributes=''  IntegratorStateMustResolveToSignalObject=off  IntegratorRTWStateStorageClass=Auto  FilterContinuousStateAttributes=''  FilterStateMustResolveToSignalObject=off  FilterRTWStateStorageClass=Auto  ParallelPVariant=InternalParameters  IdealPVariant=Disabled  IVariant=InternalParameters  DVariant=InternalParameters  IntegratorVariant=Discrete  SatVariant=Disabled  AWVariant=Passthrough  PCopyVariant=Disabled  TRVariant=Disabled  FdbkBlocksVariant=Forward  IdealPFdbkVariant=Disabled  SatFdbkVariant=Disabled  DerivativeFilterVariant=ForwardEulerFilter  NVariant=InternalParameters  NCopyVariant=Disabled  FilterICVariant=InternalICsFilter  IntegratorICVariant=InternalICs  ExternalResetVariant=Disabled  TRSumVariant=Passthrough  SumFdbkVariant=Disabled  SumVariant=Sum_PID  TsampFilterVariant=InternalTs  TsampNgainVariant=Passthrough  TsampIntegralVariant=Passthrough  ExternalSaturationOutDataTypeStr=Inherit: Same as second input  aMode=0
  cfblk5 : DiscreteFir  SampleTime=1
  cfblk6 : slpidlib/PID Controller (2DOF)  Controller=PID  Form=Parallel  TimeDomain=Discrete-time  UseExternalTs=off  SampleTime=1  IntegratorMethod=Forward Euler  FilterMethod=Forward Euler  ControllerParametersSource=internal  P=1  I=1  UseKiTs=off  D=0  N=100  UseFilter=on  b=1  c=1  TunerSelectOption=Transfer Function Based (PID Tuner App)  InitialConditionSource=internal  InitialConditionForIntegrator=0  InitialConditionForFilter=0  DifferentiatorICPrevScaledInput=0  ExternalReset=none  TrackingMode=off  Kt=1  LimitOutput=off  SatLimitsSource=internal  UpperSaturationLimit=inf  LowerSaturationLimit=-inf  LinearizeAsGain=off  AntiWindupMode=none  Kb=1  POutMin=[]  POutMax=[]  IOutMin=[]  IOutMax=[]  DOutMin=[]  DOutMax=[]  NOutMin=[]  NOutMax=[]  bOutMin=[]  bOutMax=[]  cOutMin=[]  cOutMax=[]  SumOutMin=[]  SumOutMax=[]  SaturationOutMin=[]  SaturationOutMax=[]  PParamMin=[]  PParamMax=[]  IParamMin=[]  IParamMax=[]  DParamMin=[]  DParamMax=[]  NParamMin=[]  NParamMax=[]  bParamMin=[]  bParamMax=[]  cParamMin=[]  cParamMax=[]  KbParamMin=[]  KbParamMax=[]  KtParamMin=[]  KtParamMax=[]  KbOutMin=[]  KbOutMax=[]  KtOutMin=[]  KtOutMax=[]  IntegratorOutMin=[]  IntegratorOutMax=[]  FilterOutMin=[]  FilterOutMax=[]  SumI1OutMin=[]  SumI1OutMax=[]  SumI2OutMin=[]  SumI2OutMax=[]  SumI3OutMin=[]  SumI3OutMax=[]  SumI4OutMin=[]  SumI4OutMax=[]  SumDOutMin=[]  SumDOutMax=[]  Sum1OutMin=[]  Sum1OutMax=[]  Sum2OutMin=[]  Sum2OutMax=[]  Sum3OutMin=[]  Sum3OutMax=[]  DifferentiatorOutMin=[]  DifferentiatorOutMax=[]  FilterDiffOutCoefMin=[]  FilterDiffOutCoefMax=[]  ReciprocalOutMin=[]  ReciprocalOutMax=[]  SumDenOutMin=[]  SumDenOutMax=[]  SumNumOutMin=[]  SumNumOutMax=[]  DivideOutMin=[]  DivideOutMax=[]  UdiffTsProdOutMin=[]  UdiffTsProdOutMax=[]  NTsProdOutMin=[]  NTsProdOutMax=[]  UintegralTsProdOutMin=[]  UintegralTsProdOutMax=[]  UngainTsProdOutMin=[]  UngainTsProdOutMax=[]  IntegratorContinuousStateAttributes=''  IntegratorStateMustResolveToSignalObject=off  IntegratorRTWStateStorageClass=Auto  FilterContinuousStateAttributes=''  FilterStateMustResolveToSignalObject=off  FilterRTWStateStorageClass=Auto  ParallelPVariant=InternalParameters  IdealPVariant=Disabled  IVariant=InternalParameters  DVariant=InternalParameters  bVariant=InternalParameters  cVariant=InternalParameters  IntegratorVariant=Discrete  SatVariant=Disabled  AWVariant=Passthrough  PCopyVariant=Disabled  TRVariant=Disabled  FdbkBlocksVariant=Forward  IdealPFdbkVariant=Disabled  SatFdbkVariant=Disabled  DerivativeFilterVariant=ForwardEulerFilter  NVariant=InternalParameters  NCopyVariant=Disabled  FilterICVariant=InternalICsFilter  IntegratorICVariant=InternalICs  ExternalResetVariant=Disabled  TRSumVariant=Passthrough  SumFdbkVariant=Disabled  SumVariant=Sum_PID  TsampFilterVariant=InternalTs  TsampNgainVariant=Passthrough  TsampIntegralVariant=Passthrough  ExternalSaturationOutDataTypeStr=Inherit: Same as second input
      settings: SourceProductBaseCode=SL
  cfblk7 : Rounding
  cfblk8 : Bias  Bias=[539773986.214958]  SaturateOnIntegerOverflow=off
  cfblk9 : Math  Operator=hypot
  cfblk2 : Outport
  wires:
  cfblk13/1 -> cfblk8/1
  cfblk5/1 -> cfblk10/1
  cfblk8/1 -> cfblk12/1
  cfblk3/1 -> cfblk4/1
  cfblk17/1 -> cfblk10/2
  cfblk1/1 -> cfblk11/1
  cfblk12/1 -> cfblk6/1
  cfblk14/1 -> cfblk6/2
  cfblk15/1 -> cfblk11/2
  cfblk9/1 -> cfblk2/1
  cfblk4/1 -> cfblk9/1
  cfblk11/1 -> cfblk9/2
  cfblk16/1 -> cfblk7/1
  cfblk6/1 -> cfblk5/1
  cfblk10/1 -> cfblk3/1

== system sampleModel106/cfblk84/cfblk5/cfblk13/cfblk9 ==
  cfblk1 : Inport
  cfblk11 : Inport  Port=2
  cfblk12 : Inport  Port=3
  cfblk10 : Constant  Value=[946467125.255093]  SampleTime=1
  cfblk13 : Delay  SampleTime=1
  cfblk3 : Delay  DelayLengthSource=Input port  SampleTime=1
      settings: InputPortMap=u0,p1
  cfblk4 : ComplexToRealImag
  cfblk5 : Sum
  cfblk6 : Product  Inputs=*
  cfblk7 : UnaryMinus
  cfblk8 : ComplexToRealImag
  cfblk9 : Constant  Value=[828033585.409103]  SampleTime=1
  cfblk2 : Outport
  wires:
  cfblk5/1 -> cfblk8/1
  cfblk6/1 -> cfblk7/1
  cfblk7/1 -> cfblk4/1
  cfblk4/1 -> cfblk3/1
  cfblk9/1 -> cfblk2/1
  cfblk10/1 -> cfblk6/1
  cfblk8/1 -> cfblk3/2
  cfblk1/1 -> cfblk5/2
  cfblk8/2 -> cfblk13/1
  cfblk13/1 -> cfblk5/1

== system sampleModel106/cfblk84/cfblk6/cfblk5/cfblk10 ==
  cfblk1 : Inport
  cfblk12 : Inport  Port=2
  cfblk10 : Constant  Value=[258169143.590964]  SampleTime=1
  cfblk11 : Constant  Value=[112736747.203795]  SampleTime=1
  cfblk16 : Delay  SampleTime=1
  cfblk17 : Delay  SampleTime=1
  cfblk3 : Delay  SampleTime=1
  cfblk4 : Sum  Inputs=|++
  cfblk5 : Squeeze
  cfblk6 : Bias  Bias=[159710015.156074]  SaturateOnIntegerOverflow=off
  cfblk7 : Assignment  DiagnosticForDimensions=Warning  IndexOptions=Index vector (dialog)  Indices=1  OutputSizes=1
  cfblk8 : Trigonometry
  cfblk9 : Sum  Inputs=+-
  cfblk2 : Outport
  cfblk13 : Outport  Port=2
  cfblk14 : Outport  Port=3
  cfblk15 : Outport  Port=4
  wires:
  cfblk12/1 -> cfblk13/1
  cfblk7/1 -> cfblk8/1
  cfblk8/1 -> cfblk3/1
  cfblk11/1 -> cfblk14/1, cfblk9/2
  cfblk10/1 -> cfblk15/1, cfblk4/2
  cfblk4/1 -> cfblk5/1
  cfblk5/1 -> cfblk6/1
  cfblk6/1 -> cfblk9/1, cfblk17/1
  cfblk1/1 -> cfblk7/2
  cfblk9/1 -> cfblk2/1
  cfblk3/1 -> cfblk16/1
  cfblk16/1 -> cfblk7/1
  cfblk17/1 -> cfblk4/1

== system sampleModel106/cfblk84/cfblk6/cfblk5/cfblk11 ==
  cfblk1 : Inport
  cfblk12 : Inport  Port=2
  cfblk13 : Inport  Port=3
  cfblk14 : Inport  Port=4
  cfblk10 : Constant  Value=[-789777432.078425]  SampleTime=1
  cfblk11 : Constant  Value=[-572343063.829184]  SampleTime=1
  cfblk17 : Delay  SampleTime=1
  cfblk18 : Delay  SampleTime=1
  cfblk3 : simulink/Discrete/Transfer Fcn Real Zero  ZeroZ=0.75  ICPrevInput=0.0  DoSatur=off
      settings: SourceProductBaseCode=SL
  cfblk4 : Delay  DelayLengthSource=Input port  SampleTime=1
      settings: InputPortMap=u0,p1
  cfblk5 : Polyval  Coefs=[ +2.081618890e-019, -1.441693666e-014, +4.719686976e-010, -8.536869453e-006, +1.621573104e-001, -8.087801117e+001 ]
  cfblk6 : Signum
  cfblk7 : Sum  Inputs=+-
  cfblk8 : Sin  TimeSource=Use external signal  SampleTime=0
  cfblk9 : MinMax  Function=max  Inputs=3
  cfblk2 : Outport
  cfblk15 : Outport  Port=2
  cfblk16 : Outport  Port=3
  wires:
  cfblk5/1 -> cfblk8/1
  cfblk12/1 -> cfblk7/1
  cfblk8/1 -> cfblk2/1
  cfblk1/1 -> cfblk16/1
  cfblk13/1 -> cfblk4/1
  cfblk10/1 -> cfblk3/1
  cfblk4/1 -> cfblk17/1, cfblk18/1
  cfblk11/1 -> cfblk6/1
  cfblk6/1 -> cfblk7/2
  cfblk14/1 -> cfblk15/1
  cfblk7/1 -> cfblk5/1
  cfblk3/1 -> cfblk9/2
  cfblk9/1 -> cfblk4/2
  cfblk17/1 -> cfblk9/1
  cfblk18/1 -> cfblk9/3

== system sampleModel106/cfblk84/cfblk6/cfblk5/cfblk18 ==
  cfblk1 : Inport
  cfblk8 : Inport  Port=2
  Action Port : ActionPort  ActionPortLabel=if(u1 >= 0)
  cfblk3 : ComplexToMagnitudeAngle
  cfblk4 : ComplexToRealImag
  cfblk5 : Product  Inputs=**
  cfblk6 : Constant  Value=[585746345.354594]  SampleTime=1
  cfblk7 : Constant  Value=[851997559.877680]  SampleTime=1
  cfblk2 : Outport
  cfblk9 : Outport  Port=2
  wires:
  cfblk7/1 -> cfblk4/1
  cfblk1/1 -> cfblk2/1
  cfblk6/1 -> cfblk5/1
  cfblk3/1 -> cfblk5/2
  cfblk8/1 -> cfblk3/1
  cfblk3/2 -> cfblk9/1

== system sampleModel106/cfblk84/cfblk6/cfblk5/cfblk19 ==
  cfblk1 : Inport
  cfblk6 : Inport  Port=2
  cfblk7 : Inport  Port=3
  Action Port : ActionPort  ActionPortLabel=else
  cfblk3 : DiscreteZeroPole  Poles=[0 0.5]  Gain=1  SampleTime=-1
  cfblk4 : Sin  TimeSource=Use external signal  SampleTime=0
  cfblk5 : Constant  Value=[789323051.219469]  SampleTime=1
  cfblk9 : Delay
  cfblk2 : Outport
  cfblk8 : Outport  Port=2
  wires:
  cfblk1/1 -> cfblk8/1
  cfblk6/1 -> cfblk2/1
  cfblk3/1 -> cfblk4/1
  cfblk4/1 -> cfblk9/1
  cfblk9/1 -> cfblk3/1

== system sampleModel106/cfblk84/cfblk6/cfblk5/cfblk9 ==
  cfblk1 : Inport
  cfblk3 : DotProduct  OutDataTypeStr=Inherit: Inherit via internal rule
  cfblk4 : Product
  cfblk5 : Sin  TimeSource=Use external signal  SampleTime=0
  cfblk8 : Delay  SampleTime=1
  cfblk2 : Outport
  cfblk6 : Outport  Port=2
  cfblk7 : Outport  Port=3
  wires:
  cfblk3/1 -> cfblk2/1, cfblk6/1, cfblk5/1
  cfblk5/1 -> cfblk7/1, cfblk4/1, cfblk4/2
  cfblk1/1 -> cfblk3/2
  cfblk4/1 -> cfblk8/1
  cfblk8/1 -> cfblk3/1
